simulink model "microgrid_WithBESS"  (R2023a)
settings: Solver=ode23t  StartTime=0.0  StopTime=86000  RelTol=1e-3
PreLoadFcn:
  | addpath('Resources')
InitFcn:
  | initialConditions();
values from neighbouring files (symbols this model uses):
  battEnergy = 3.6e6*BattCap    (= 2059200000)    [initialConditions.m]
  optTime = timeOptimize*60    (= 300)    [initialConditions.m]
libraries: simulink x8, spsThreePhaseDynamicLoadLib x3, spsPower3phPhasorLib x3, spsThreePhaseVIMeasurementLib x3, spsThreePhaseBreakerLib x3, spsThreePhaseSourceLib x2, spsThreePhasePISectionLineLib x1, spsThreePhaseSeriesRLCLoadLib x1, powerlib_meascontrol x1, powerlib x1, spsFrequencyPhasorLib x1, spsSequenceAnalyzerPhasorLib x1
settings Model: Creator=jlesage  LastModifiedBy=KeronDenny
settings SolverCC: AlgebraicLoopSolver=TrustRegion
settings DataIOCC: ReturnWorkspaceOutputs=off
settings DebuggingCC: PregeneratedLibrarySubsystemCodeDiagnostic=none  ArithmeticOperatorsInVariantConditions=warning
settings ModelReferenceCC: EnableRefExpFcnMdlSchedulingChecks=on
settings SFSimCC: SimUseLocalCustomCode=off  CustomCodeUndefinedFunction=UseInterfaceOnly
settings RTWCC: RTWUseLocalCustomCode=off

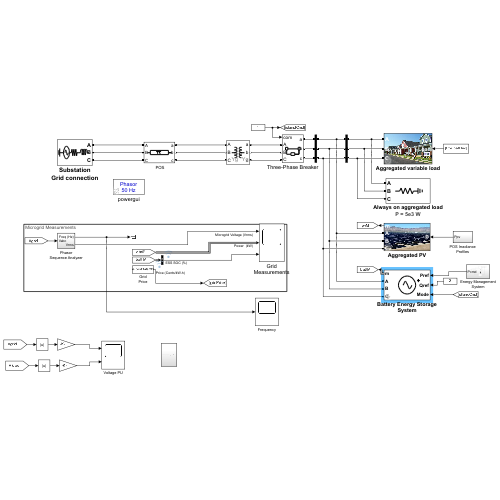
[thumbnail: Simulink's stored preview of the top-level diagram]
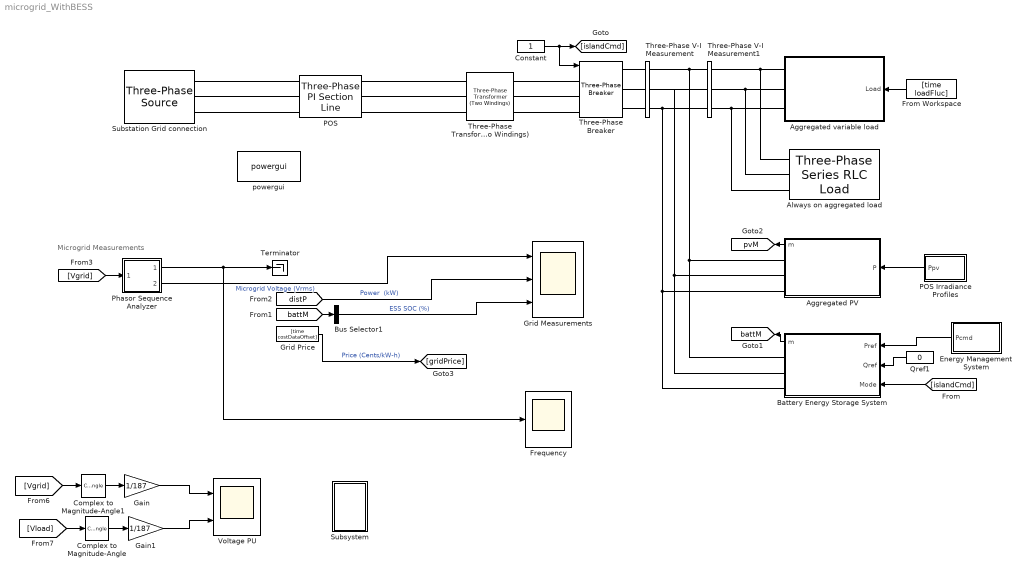
== system microgrid_WithBESS ==
  note: Microgrid Measurements
  " POS " : spsThreePhasePISectionLineLib/Three-Phase PI Section Line  LConnTagsString=a|b|c  RConnTagsString=A|B|C  Length=1.18  Frequency=50  Resistances=[60.9 0.001]  Inductances="[3.52e-2  3.483e-3]"  Capacitances="[ 11.09729e-09   4.8118e-09]"
  Aggregated PV : Subsystem  mask(Grid-Connected PV Array (PQ Model)){Vn=230, Fn=50, P0=400e3}
      mask prompts: Vn "Nominal L-L Voltage [Vrms]"; Fn "Nominal Frequency [Hz]"; P0 "Initial Power [W]"
      mask help:
      | This block models a grid-connected solar array using the Three-Phase Dynamic Load block. This is a system-level model that does not contain any power electronics, but is useful for load flow, phasor, and hybrid phasor-EMT simulations. The input to this block is the power output of the grid connected PV array, not irradiance.
      |
      | For more detailed PV models, consider the PV Array block in the Renewables library. Consider using this PQ Model to perform load flow studies and switch to a more detailed model when full EMT studies are required.
      |
      | Note: The array power must be specified for use for Load Flow analysis.
      mask init:
      | % P0 = Irr0*TotalArea*Efficiency/100;
      | P0 = -P0;
      mask Display:
      | image(imread('PV_Farm.jpg'))
      | color('white')
      | port_label('input',1,'P')
      | port_label('output',1,'m')
      | port_label('Rconn',1,'A')
      | port_label('Rconn',2,'B')
      | port_label('Rconn',3,'C')
  Aggregated variable load : Subsystem  mask(Variable Load (PQ Model)){Vn=230, Fn=50, PF=1, Load0=10e3}
      mask prompts: Vn "Nominal L-L Voltage [Vrms]"; Fn "Nominal Frequency [Hz]"; PF "Power Factor [0 to 1]"; Load0 "Initial Load [W]"
      mask help:
      | The Variable Load block is a lumped approximation for a distribution feeder. For non-unity power factor loads, the input (active power) is scaled accordingly to generate a desired load.
      |
      | Note: The initial input load must be specified for use for Load Flow analysis.
      mask init:
      | P0 = Load0;
      | Q0 = Load0*sqrt(1/PF^2-1);
      mask Display:
      | image(imread('Residential.jpg'))
      | color('white')
      | port_label('input',1,'Load')
      | port_label('Rconn',1,'A')
      | port_label('Rconn',2,'B')
      | port_label('Rconn',3,'C')
  Always on aggregated load : spsThreePhaseSeriesRLCLoadLib/Three-Phase Series RLC Load  LConnTagsString=A|B|C  Configuration=Y (grounded)  NominalVoltage=230  Vabc=[1e3 1e3 1e3]  Vabcp=[1e3 1e3 1e3]  NominalFrequency=50  UnbalancedPower=off  ActivePower=5e3  InductivePower=0  CapacitivePower=0  Pabc=[10e3 9e3 11e3]  QLabc=[100 90 110]  QCabc=[100 90 110]  Pabcp=[10e3 9e3 11e3]  QLabcp=[100 90 110]  QCabcp=[100 90 110]  Measurements=None  LoadType=constant Z
      settings: AttributesFormatString=P = %<ActivePower> W
  Battery Energy Storage System : Subsystem  mask(Grid-connected Energy Storage (PQ Model)){SimMode=Phasor, Vn=230, Fn=50, PnomkW=143, kWh_Rated=572, Efficiency=96, LimitVec=[79 21], RechargeSOC=12, Precharge=100, autoRecharge=on, Initial_kWh_pc=21, PQvec=[400e3 0]}
      mask prompts: SimMode "Simulation Mode"; Vn "Nominal L-L Voltage [Vrms]"; Fn "Nominal Frequency [Hz]"; PnomkW "Rated Power [kW]"; kWh_Rated "Rated Capacity [kWh]"; Efficiency "Overall System Efficiency [%]"; LimitVec "Upper/Lower Charge Limits [%]"; RechargeSOC "SOC to Recharge [%]"; Precharge "Recharge Rate [% of Rated Power]"; autoRecharge "Enable Auto-Recharge"; Initial_kWh_pc "Initial State-of-Charge [0-100%]"; PQvec "Initial Active/Reactive Cmds"
      mask help:
      | The energy storage block models a generic grid-connected energy storage system (ESS), most commonly a battery system. This is a system-level model that does not contain any power electronics, but is useful for load flow, phasor, and hybrid phasor-EMT simulations. The inputs to this block are the commanded active and reactive power of the ESS. The ESS is assumed to have four quadrent operation. The Mode Input dictates what high-level operation the ESS has: current control (Mode = 1) or voltage control (Mode = 0). Current control is ideal for a grid connected system where you need to specify P,Q commands. Voltage control is necessary if the ESS will be the only system supporting the microgrid in islanded mode.
      |
      | For more detailed ESS models, consider the battery block in the Drives library. Consider using this PQ Model to perform load flow studies and switch to a more detailed model when full EMT studies or more advanced controls are required.
      |
      | Note: The initial active/reactive power commands must be specified for use for Load Flow analysis.
      mask init:
      | % Calculate Initial Conditions
      | Pnom = PnomkW*1e3;
      | P0 = -PQvec(1);  Q0 = -PQvec(2);
      | if abs(P0) > Pnom
      |     P0 = sign(P0)*Pnom;
      | end
      | 
      | % Calculate Q0 given Reactive Power Capability Curve
      | Qlim = sqrt(Pnom^2 - P0^2);
      | if Qlim > abs(Q0)
      |     Q0 = sign(Q0)*Qlim;
      | end
      | 
      | UpChrgLim = LimitVec(1);
      | LowChrgLim = LimitVec(2);
      | if Initial_kWh_pc > UpChrgLim && P0 < 0
      |     P0 = 0; Q0 = 0;
      | elseif Initial_kWh_pc < LowChrgLim && P0 > 0
      |     P0 = 0; Q0 = 0;
      | end
      | 
      | simulationStatus =  get_param(bdroot,'SimulationStatus');
      | 
      | % The active variant can only be modified at edit-time or very early during
      | % the simulink compile stage. 
      | if any(strcmp(simulationStatus, {'stopped'}))
      | 
      | blk = [gcb '/Power Measures'];
      | if strcmp(SimMode,'Phasor')
      |     set_param(blk,'OverrideUsingVariant','Phasor');
      | else
      |     set_param(blk,'OverrideUsingVariant','EMT');
      | end
      | 
      | 
      | end
      mask TypeOptions SimMode: Electromagnetic Transient (EMT) | Phasor
      mask DialogControl Container7 Prompt: Grid Connection Properties
      mask DialogControl Container11 Prompt: Charge/Discharge Controls
      mask DialogControl Container12 Prompt: Initial Conditions
      mask Display: plot(-80,-50,80,50,[0,9,18,24,29,30,29,24,18,9,0,-9,-18,-24,-29,-30,-29,-24,-18,-9,0],[30,29,24,18,9,0,-9,-18,-24,-29,-30,-29,-24,-18,-9,0,9,18,24,29,30],[-50],[0],[50],[0],[45 35 40 40 40],[15 15 15 20 10],[1 2 3 4 5 6 7 8 9 10 11 12 13 14 15 16 17 18 19 20 21].*1.5-15,[0,9,18,24,29,30,29,24,18,9,0,-9,-18,-24,-29,-30,-29,-24,-18,-9,0]./2.4)
  Bus Selector1 : BusSelector  OutputSignals=SOC (%)  OutputAsBus=on
  Complex to Magnitude-Angle : ComplexToMagnitudeAngle  Output=Magnitude
  Complex to Magnitude-Angle1 : ComplexToMagnitudeAngle  Output=Magnitude
  Constant : Constant
  Energy Management System : Subsystem
  Frequency : Scope
  From Workspace : FromWorkspace  VariableName=[time loadFluc]
  Gain : Gain  Gain=1/187
  Gain1 : Gain  Gain=1/187
  Grid Measurements : Scope  NumInputPorts=3
  Grid Price : FromWorkspace  VariableName=[time costDataOffset]
  POS Irradiance Profiles : Subsystem
  Phasor Sequence Analyzer : Subsystem
  Qref1 : Constant  Value=0
  Substation Grid connection : spsThreePhaseSourceLib/Three-Phase Source  InternalConnection=Yg  VoltagePhases=off  Voltage=(11000)*1  PhaseAngle=0.071468  Voltage_phases=[25e3 25e3 25e3]/sqrt(3)  PhaseAngles_phases=[0 -120 +120]  Frequency=50  NonIdealSource=on  SpecifyImpedance=on  Resistance=0.8929  Inductance=16.58e-3  ShortCircuitLevel=200e3  BaseVoltage=230  XRratio=0.07  BusType=swing  Pref=10e3  Qref=0  Prefabc=[10e3, 10e3, 10e3]  Qrefabc=[0, 0, 0]  Qmin=-inf  Qmax=inf
  Subsystem : Subsystem
  Terminator : Terminator
  Three-Phase Transformer (Two Windings) : spsThreePhaseTransformerTwoWindingsLib/Three-Phase Transformer (Two Windings)  Winding1Connection=Yg  Winding2Connection=Yg  CoreType=Three single-phase transformers  SetSaturation=off  Hysteresis=off  DataFile='hysteresis'  SetInitialFlux=off  Measurements=None  UNITS=pu  NominalPower=[200e3, 50 ]  Winding1=[ 11e3 , 0.002 , 0.08 ]  Winding2=[ 230 , 0.002 , 0.08 ]  Rm=500  Lm=500  L0=0.5  Saturation=[ 0,0 ; 0.0024,1.2 ; 1.0,1.52 ]  InitialFluxes=[ 0.8 , -0.8 , 0.7 ]  BreakLoop=off  DiscreteSolver=Trapezoidal iterative  DataType=off  TransfoNumber=1
  Three-Phase V-I Measurement : spsThreePhaseVIMeasurementLib/Three-Phase V-I Measurement  VoltageMeasurement=phase-to-ground  SetLabelV=on  LabelV=Vgrid  Vpu=off  VpuLL=off  CurrentMeasurement=yes  SetLabelI=on  LabelI=Igrid  Ipu=off  Pbase=100e6  Vbase=500e3  OutputType=Complex  PhasorSimulation=on  PSBequivalent=0
  Three-Phase V-I Measurement1 : spsThreePhaseVIMeasurementLib/Three-Phase V-I Measurement  VoltageMeasurement=phase-to-ground  SetLabelV=on  LabelV=Vload  Vpu=off  VpuLL=off  CurrentMeasurement=yes  SetLabelI=on  LabelI=Iload  Ipu=off  Pbase=100e6  Vbase=500e3  OutputType=Complex  PhasorSimulation=on  PSBequivalent=0
  Three-Phase Breaker : spsThreePhaseBreakerLib/Three-Phase Breaker  InitialState=closed  SwitchA=on  SwitchB=on  SwitchC=on  SwitchTimes="[1/60  5/60]"  External=on  BreakerResistance=0.01  SnubberResistance=1e6  SnubberCapacitance=inf  Measurements=None
  Voltage PU : Scope  NumInputPorts=2
  powergui : sps_lib/powergui  Priority=1  SimulationMode=Phasor  SampleTime=1e-4  frequency=50  Iterations=50  frequencyindice=50  Pbase=100e6  ErrMax=0.0001  UnitsV=kV  UnitsW=MW  buscounter=3  FunctionMessages=off  echomessages=off  EnableUseOfTLC=off  CurrentSourceSwitches=off  DisableSnubberDevices=off  DisableRonSwitches=off  DisableVfSwitches=off  DisplayEquations=off  AutomaticDiscreteSolvers=off  SolverType=Tustin/Backward Euler (TBE)  Interpol=off  ExternalGateDelay=off  methode=off  Ts=100  x0status=blocks  SPID=on  SwTol=0  HookPort=off  NonlinearTolerance=0  nMaxIteration=15  ContinueOnMaxIteration=off  RestoreLinks=warning  ResistiveCurrentMeasurement=off  Frange=[0:2:500]  Ylog=off  Xlog=on  ShowGrid=off  save=off  variable=ZData  structure=0  ZoomFFT=off  StartTime=0.0  cycles=1  DisplayStyle=1  fundamental=60  FreqAxis=off  MaxFrequency=1000  frequencyindicesteady=1  RmsSteady=1  display=off
  tag scope: battM=global, pvM=global
  wires:
  Qref1/1 -> Battery Energy Storage System/2(Qref)
  Battery Energy Storage System/1(m) -> [battM]
  Aggregated PV/1(m) -> [pvM]
  [Vgrid] -> Phasor Sequence Analyzer/1(Vabc)
  [islandCmd] -> Battery Energy Storage System/3(Mode)
  Constant/1 -> [islandCmd], Three-Phase Breaker/1
  [distP] -> Grid Measurements/2  "Power  (kW)"
  Phasor Sequence Analyzer/2(Vrms) -> Grid Measurements/1  "Microgrid Voltage (Vrms)"
  [battM] -> Bus Selector1/1
  Phasor Sequence Analyzer/1(Freq (Hz)) -> Terminator/1, Frequency/1
  Grid Price/1 -> [gridPrice]  "Price (Cents/kW-h)"
  [Vload] -> Complex to Magnitude-Angle/1
  [Vgrid] -> Complex to Magnitude-Angle1/1
  Complex to Magnitude-Angle/1 -> Gain1/1
  Complex to Magnitude-Angle1/1 -> Gain/1
  Gain/1 -> Voltage PU/1
  Gain1/1 -> Voltage PU/2
  Bus Selector1/1 -> Grid Measurements/3  "ESS SOC (%)"
  Energy Management System/1(Pcmd) -> Battery Energy Storage System/1(Pref)
  POS Irradiance Profiles/1(Ppv) -> Aggregated PV/1(P)
  From Workspace/1 -> Aggregated variable load/1(Load)
  connections:
  " POS "/RConn1 -- Three-Phase Transformer (Two Windings)/LConn1
  " POS "/RConn2 -- Three-Phase Transformer (Two Windings)/LConn2
  " POS "/RConn3 -- Three-Phase Transformer (Two Windings)/LConn3
  Three-Phase Transformer (Two Windings)/RConn1 -- Three-Phase Breaker/LConn1
  Three-Phase Transformer (Two Windings)/RConn2 -- Three-Phase Breaker/LConn2
  Three-Phase Transformer (Two Windings)/RConn3 -- Three-Phase Breaker/LConn3
  Always on aggregated load/LConn2 -- Aggregated variable load/RConn2 -- Three-Phase V-I Measurement1/RConn2
  Three-Phase V-I Measurement/RConn3 -- Three-Phase V-I Measurement1/LConn3 -- Battery Energy Storage System/RConn3 -- Aggregated PV/RConn3
  Three-Phase Breaker/RConn1 -- Three-Phase V-I Measurement/LConn1
  Three-Phase Breaker/RConn2 -- Three-Phase V-I Measurement/LConn2
  Three-Phase Breaker/RConn3 -- Three-Phase V-I Measurement/LConn3
  Always on aggregated load/LConn1 -- Aggregated variable load/RConn1 -- Three-Phase V-I Measurement1/RConn1
  Three-Phase V-I Measurement/RConn1 -- Three-Phase V-I Measurement1/LConn1 -- Battery Energy Storage System/RConn1 -- Aggregated PV/RConn1
  Battery Energy Storage System/RConn2 -- Three-Phase V-I Measurement/RConn2 -- Three-Phase V-I Measurement1/LConn2 -- Aggregated PV/RConn2
  Always on aggregated load/LConn3 -- Aggregated variable load/RConn3 -- Three-Phase V-I Measurement1/RConn3
  Substation Grid connection/RConn1 -- " POS "/LConn1
  Substation Grid connection/RConn2 -- " POS "/LConn2
  Substation Grid connection/RConn3 -- " POS "/LConn3

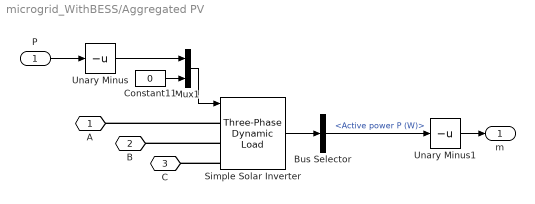
== system microgrid_WithBESS/Aggregated PV ==
  P : Inport
  Bus Selector : BusSelector  OutputSignals=Active power P (W)
  Constant11 : Constant  Value=0
  Mux1 : Mux  Inputs=2
  Simple Solar Inverter : spsThreePhaseDynamicLoadLib/Three-Phase Dynamic Load  NominalVoltage=[Vn Fn]  ActiveReactivePowers=[-250000 -3.38813e-13]  PositiveSequence=[0.999844 -0.0038635]  ExternalControl=on  NpNq=[1.3 2]  TimeConstants="[0  0  0  0]"  MinimumVoltage=0.7  Tfilter=1e-2  LoadFlowParameters=[4,0,0,0,0]
      settings: LibrarySourceBlock=|
      | sps_lib/Passives/Three-Phase
      | Dynamic Load
  Unary Minus : UnaryMinus
  Unary Minus1 : UnaryMinus
  A : PMIOPort  Side=Right
  B : PMIOPort  Port=2  Side=Right
  C : PMIOPort  Port=3  Side=Right
  m : Outport  VectorParamsAs1DForOutWhenUnconnected=off
  wires:
  P/1 -> Unary Minus/1
  Unary Minus/1 -> Mux1/1
  Mux1/1 -> Simple Solar Inverter/1
  Constant11/1 -> Mux1/2
  Simple Solar Inverter/1 -> Bus Selector/1
  Bus Selector/1 -> Unary Minus1/1  "<Active power P (W)>"
  Unary Minus1/1 -> m/1
  connections:
  Simple Solar Inverter/LConn2 -- B/RConn1
  Simple Solar Inverter/LConn3 -- C/RConn1
  Simple Solar Inverter/LConn1 -- A/RConn1

== system microgrid_WithBESS/Aggregated variable load ==
  Load : Inport
  Dynamic Load Control : Subsystem
  Simple Three-Phase Load : spsThreePhaseDynamicLoadLib/Three-Phase Dynamic Load  NominalVoltage=[Vn Fn]  ActiveReactivePowers=[200000 45883.1]  PositiveSequence=[0.999844 -0.0038635]  ExternalControl=on  NpNq=[1.3 2]  TimeConstants="[0  0  0  0]"  MinimumVoltage=0.7  Tfilter=1e-2  LoadFlowParameters=[4,0,0,0,0]
      settings: LibrarySourceBlock=|
      | sps_lib/Passives/Three-Phase
      | Dynamic Load
  Terminator : Terminator
  A : PMIOPort  Side=Right
  B : PMIOPort  Port=2  Side=Right
  C : PMIOPort  Port=3  Side=Right
  wires:
  Simple Three-Phase Load/1 -> Terminator/1
  Load/1 -> Dynamic Load Control/1(P0)
  Dynamic Load Control/1(PQ) -> Simple Three-Phase Load/1
  connections:
  Simple Three-Phase Load/LConn1 -- A/RConn1
  Simple Three-Phase Load/LConn3 -- C/RConn1
  Simple Three-Phase Load/LConn2 -- B/RConn1

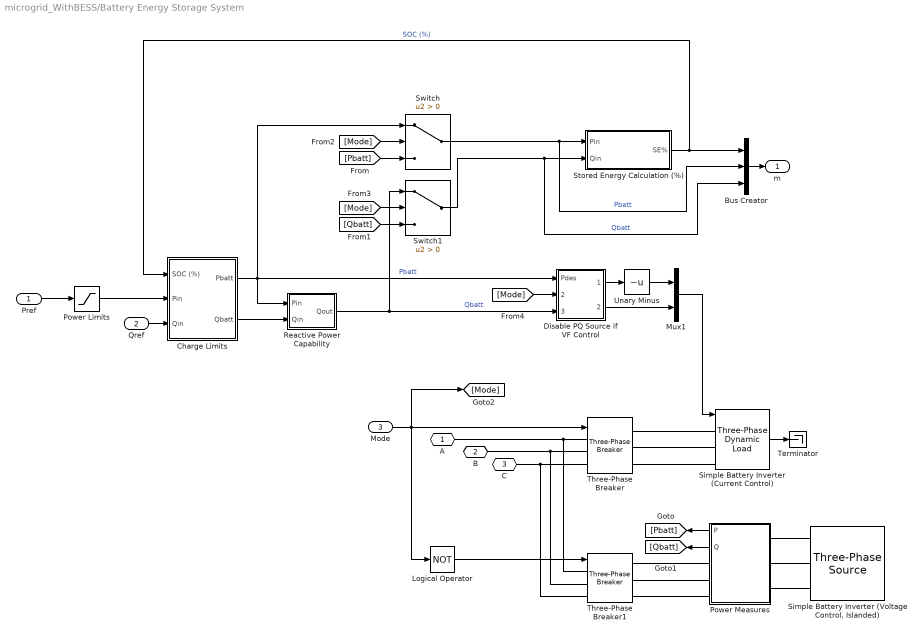
== system microgrid_WithBESS/Battery Energy Storage System ==
  Pref : Inport
  Qref : Inport  Port=2
  Mode : Inport  Port=3
  Bus Creator : BusCreator  Inputs=3
  Charge Limits : Subsystem
  Disable PQ Source if VF Control : Subsystem
  Logical Operator : Logic  Operator=NOT  AllPortsSameDT=off  OutDataTypeStr=boolean
  Mux1 : Mux  Inputs=2
  Power Limits : Saturate  UpperLimit=Pnom  LowerLimit=-Pnom
  Power Measures : Subsystem  Variant=on  VariantControlMode=label  LabelModeActiveChoice=Phasor
  Reactive Power Capability : Subsystem
  Simple Battery Inverter (Current Control) : spsThreePhaseDynamicLoadLib/Three-Phase Dynamic Load  NominalVoltage=[Vn Fn]  ActiveReactivePowers=[-100e3 -3.38813e-13]  PositiveSequence=[0.999844 -0.0038635]  ExternalControl=on  NpNq=[1.3 2]  TimeConstants="[0  0  0  0]"  MinimumVoltage=0.7  Tfilter=1e-2  LoadFlowParameters=[4,0,0,0,0]
      settings: LibrarySourceBlock=|
      | sps_lib/Passives/Three-Phase
      | Dynamic Load
  "Simple Battery Inverter (Voltage Control, Islanded)" : spsThreePhaseSourceLib/Three-Phase Source  InternalConnection=Yg  VoltagePhases=off  Voltage=Vn  PhaseAngle=0  Voltage_phases=[25e3 25e3 25e3]/sqrt(3)  PhaseAngles_phases=[0 -120 +120]  Frequency=Fn  NonIdealSource=off  SpecifyImpedance=off  Resistance=0.8929  Inductance=16.58e-3  ShortCircuitLevel=100e6  BaseVoltage=25e3  XRratio=7  BusType=swing  Pref=10e3  Qref=0  Prefabc=[10e3, 10e3, 10e3]  Qrefabc=[0, 0, 0]  Qmin=-inf  Qmax=inf
  Stored Energy Calculation (%) : Subsystem
  Switch : Switch  Criteria=u2 > Threshold  SaturateOnIntegerOverflow=off  InputSameDT=off
  Switch1 : Switch  Criteria=u2 > Threshold  SaturateOnIntegerOverflow=off  InputSameDT=off
  Terminator : Terminator
  Three-Phase Breaker : spsThreePhaseBreakerLib/Three-Phase Breaker  InitialState=closed  SwitchA=on  SwitchB=on  SwitchC=on  SwitchTimes="[1/60  5/60]"  External=on  BreakerResistance=0.01  SnubberResistance=1e6  SnubberCapacitance=inf  Measurements=None
  Three-Phase Breaker1 : spsThreePhaseBreakerLib/Three-Phase Breaker  InitialState=open  SwitchA=on  SwitchB=on  SwitchC=on  SwitchTimes="[1/60  5/60]"  External=on  BreakerResistance=0.01  SnubberResistance=1e6  SnubberCapacitance=inf  Measurements=None
  Unary Minus : UnaryMinus
  A : PMIOPort  Side=Right
  B : PMIOPort  Port=2  Side=Right
  C : PMIOPort  Port=3  Side=Right
  m : Outport  VectorParamsAs1DForOutWhenUnconnected=off
  wires:
  Charge Limits/2(Qbatt) -> Reactive Power Capability/2(Qin)
  Qref/1 -> Charge Limits/3(Qin)
  Power Limits/1 -> Charge Limits/2(Pin)
  Stored Energy Calculation (%)/1(SE%) -> Bus Creator/1, Charge Limits/1(SOC (%))  "SOC (%)"
  Bus Creator/1 -> m/1
  Pref/1 -> Power Limits/1
  Simple Battery Inverter (Current Control)/1 -> Terminator/1
  Mux1/1 -> Simple Battery Inverter (Current Control)/1
  Unary Minus/1 -> Mux1/1
  Logical Operator/1 -> Three-Phase Breaker1/1
  Mode/1 -> [Mode], Logical Operator/1, Three-Phase Breaker/1
  Power Measures/1(P) -> [Pbatt]
  Power Measures/2(Q) -> [Qbatt]
  Switch/1 -> Bus Creator/2, Stored Energy Calculation (%)/1(Pin)  "Pbatt"
  Switch1/1 -> Bus Creator/3, Stored Energy Calculation (%)/2(Qin)  "Qbatt"
  [Mode] -> Switch/2
  [Mode] -> Switch1/2
  [Qbatt] -> Switch1/3
  [Pbatt] -> Switch/3
  Charge Limits/1(Pbatt) -> Switch/1, Reactive Power Capability/1(Pin), Disable PQ Source if VF Control/1(Pdes)  "Pbatt"
  [Mode] -> Disable PQ Source if VF Control/2(Mode)
  Reactive Power Capability/1(Qout) -> Disable PQ Source if VF Control/3(Qdes), Switch1/1  "Qbatt"
  Disable PQ Source if VF Control/1(Pbatt) -> Unary Minus/1
  Disable PQ Source if VF Control/2(Qbatt) -> Mux1/2
  connections:
  Three-Phase Breaker/RConn1 -- Simple Battery Inverter (Current Control)/LConn1
  Three-Phase Breaker/RConn2 -- Simple Battery Inverter (Current Control)/LConn2
  Three-Phase Breaker/RConn3 -- Simple Battery Inverter (Current Control)/LConn3
  Three-Phase Breaker/LConn3 -- Three-Phase Breaker1/LConn3 -- C/RConn1
  Three-Phase Breaker/LConn2 -- B/RConn1 -- Three-Phase Breaker1/LConn2
  Three-Phase Breaker/LConn1 -- A/RConn1 -- Three-Phase Breaker1/LConn1
  Power Measures/LConn1 -- "Simple Battery Inverter (Voltage Control, Islanded)"/RConn1
  Power Measures/RConn1 -- Three-Phase Breaker1/RConn1
  Power Measures/LConn2 -- "Simple Battery Inverter (Voltage Control, Islanded)"/RConn2
  Power Measures/RConn2 -- Three-Phase Breaker1/RConn2
  Power Measures/LConn3 -- "Simple Battery Inverter (Voltage Control, Islanded)"/RConn3
  Power Measures/RConn3 -- Three-Phase Breaker1/RConn3

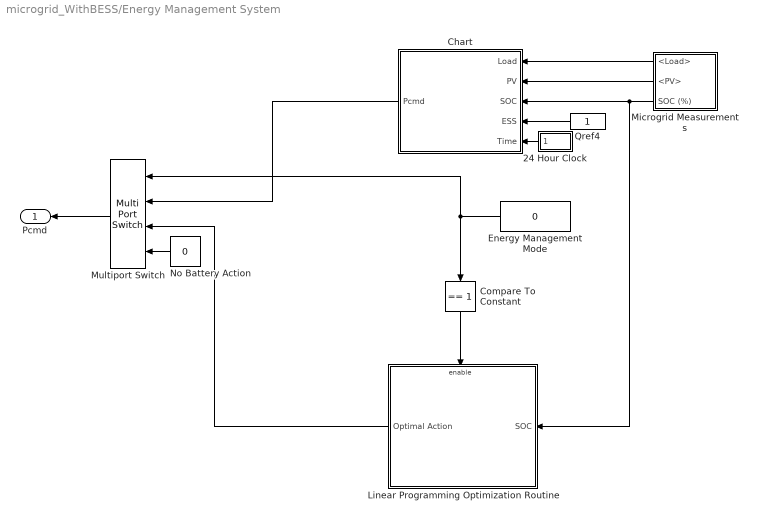
== system microgrid_WithBESS/Energy Management System ==
  24 Hour Clock : Subsystem
  Chart : Stateflow chart  TreatAsAtomicUnit=on  SystemSampleTime=360
  Compare To Constant : simulink/Logic and Bit Operations/Compare To Constant  relop===  const=1  OutDataTypeStr=boolean
  Energy Management Mode : Constant  Value=0
  Linear Programming Optimization Routine : Subsystem  TreatAsAtomicUnit=on
  Microgrid Measurements : Subsystem
  Multiport Switch : MultiPortSwitch  DataPortOrder=Zero-based contiguous  zeroidx=on  SaturateOnIntegerOverflow=off  InputSameDT=off
  No Battery Action : Constant  Value=0
  Qref4 : Constant
  Pcmd : Outport  VectorParamsAs1DForOutWhenUnconnected=off
  wires:
  Microgrid Measurements/1(<Load>) -> Chart/1(Load)
  24 Hour Clock/1(Time) -> Chart/5(Time)
  Microgrid Measurements/2(<PV>) -> Chart/2(PV)
  Microgrid Measurements/3(SOC (%)) -> Chart/3(SOC), Linear Programming Optimization Routine/1(SOC)
  Qref4/1 -> Chart/4(ESS)
  Multiport Switch/1 -> Pcmd/1
  Chart/1(Pcmd) -> Multiport Switch/2
  Energy Management Mode/1 -> Multiport Switch/1, Compare To Constant/1
  Linear Programming Optimization Routine/1(Optimal Action) -> Multiport Switch/3
  Compare To Constant/1 -> Linear Programming Optimization Routine/Enable
  No Battery Action/1 -> Multiport Switch/4

== system microgrid_WithBESS/POS Irradiance Profiles ==
  From Workspace1 : FromWorkspace  VariableName=[time cloudyPpv]
  From Workspace2 : FromWorkspace  VariableName=[time clearPpv]
  Profile Select : Constant  Value=0
  Switch : Switch  Criteria=u2 > Threshold  SaturateOnIntegerOverflow=off  InputSameDT=off
  Ppv : Outport  VectorParamsAs1DForOutWhenUnconnected=off
  wires:
  From Workspace2/1 -> Switch/1
  Profile Select/1 -> Switch/2, [PVDay]
  From Workspace1/1 -> Switch/3
  Switch/1 -> Ppv/1

== system microgrid_WithBESS/Phasor Sequence Analyzer ==
  Vabc : Inport
  Frequency (Phasor) : spsFrequencyPhasorLib/Frequency (Phasor)  Fn=50  T=0.1
      settings: LibrarySourceBlock=|
      | sps_lib/Sensors and Measurements/Frequency
      | (Phasor)
  LG to LL : Gain  Gain=sqrt(3)/sqrt(2)
  Sequence Analyzer (Phasor) : spsSequenceAnalyzerPhasorLib/Sequence Analyzer (Phasor)  seq=Positive
      settings: LibrarySourceBlock=|
      | sps_lib/Sensors and Measurements/Sequence Analyzer
      | (Phasor)
  Terminator : Terminator
  deg-to-rad : Gain  Gain=pi/180
  Freq (Hz) : Outport  VectorParamsAs1DForOutWhenUnconnected=off
  Vrms : Outport  Port=2  VectorParamsAs1DForOutWhenUnconnected=off
  wires:
  Sequence Analyzer (Phasor)/1 -> LG to LL/1
  Vabc/1 -> Sequence Analyzer (Phasor)/1
  Sequence Analyzer (Phasor)/2 -> deg-to-rad/1
  deg-to-rad/1 -> Frequency (Phasor)/1
  Frequency (Phasor)/1 -> Freq (Hz)/1
  Frequency (Phasor)/2 -> Terminator/1
  LG to LL/1 -> Vrms/1

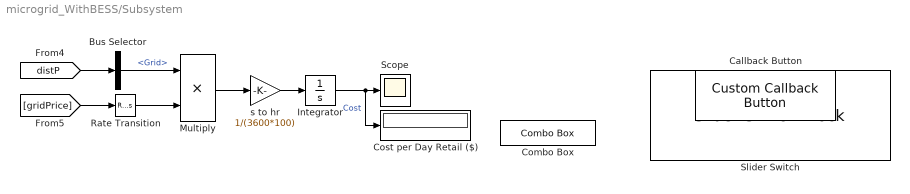
== system microgrid_WithBESS/Subsystem ==
  Bus Selector : BusSelector  OutputSignals=Grid
  Callback Button : CustomCallbackButton  Configuration="{\"components\":[{\"name\":\"BackgroundImageComponent\",\"settings\":{\"image\":{\"size\":[0,0],\"src\":\"default\",\"srcOrientation\":\"Right\"},\"position\":[0,0,1,1]}},{\"name\":\"ButtonStateComponent\",\"settings\":{\"buttonType\":\"momentary\",\"clickFcn\":\"compareCosts();\",\"onValue\":1,\"position\":[0,0,1,1],\"pressDelay\":\"500\",\"pressFcn\":\"\",\"repeatInterval\":\"0\",\"states\":[{\"horizontalAlignment\":\"center\",\"image\":{\"position\":[0,0,1,1],\"src\":\"default\",\"srcOrientation\":\"Right\"},\"label\":{\"color\":[0.01176470588,0.01176470588,0.01176470588,1],\"icon\":{\"size\":[0,0],\"src\":\"default\",\"srcOrientation\":\"Right\"},\"iconPlacement\":\"left\",\"text\":{\"content\":\"Compare Methods\"}},\"labelOffset\":[0,0],\"verticalAlignment\":\"middle\"},{\"horizontalAlignment\":\"center\",\"image\":{\"position\":[0,0,1,1],\"src\":\"default\",\"srcOrientation\":\"Right\"},\"label\":{\"color\":[0.01176470588,0.01176470588,0.01176470588,1],\"icon\":{\"size\":[0,0],\"src\":\"default\",\"srcOrientation\":\"Right\"},\"iconPlacement\":\"left\",\"text\":{\"content\":\"Compare Methods\"}},\"labelOffset\":[0,0],\"verticalAlignment\":\"middle\"},{\"horizontalAlignment\":\"center\",\"image\":{\"position\":[0,0,1,1],\"src\":\"default\",\"srcOrientation\":\"Right\"},\"label\":{\"color\":[0.01176470588,0.01176470588,0.01176470588,1],\"icon\":{\"size\":[0,0],\"src\":\"default\",\"srcOrientation\":\"Right\"},\"iconPlacement\":\"left\",\"text\":{\"content\":\"Compare Methods\"}},\"labelOffset\":[0,0],\"verticalAlignment\":\"middle\"},{\"horizontalAlignment\":\"center\",\"image\":{\"position\":[0,0,1,1],\"src\":\"default\",\"srcOrientation\":\"Right\"},\"label\":{\"color\":[0.01176470588,0.01176470588,0.01176470588,1],\"icon\":{\"size\":[0,0],\"src\":\"default\",\"srcOrientation\":\"Right\"},\"iconPlacement\":\"left\",\"text\":{\"content\":\"Compare Methods\"}},\"labelOffset\":[0,0],\"verticalAlignment\":\"middle\"}]}},{\"name\":\"ForegroundImageComponent\",\"settings\":{\"image\":{\"size\":[0,0],\"src\":\"default\",\"srcOrientation\":\"Right\"},\"isForeground\":1,\"position\":[0,0,1,1]}}],\"settings\":{\"BindingType\":\"standalone\",\"backgroundColor\":[244,244,244,1],\"backgroundOffset\":0.2,\"backgroundOpacity\":1,\"fixedAspectRatio\":\"off\",\"foregroundColor\":[0.01176470588,0.01176470588,0.01176470588,1],\"migratedFromLegacy\":true,\"useBackgroundColor\":true,\"variant\":\"callback\",\"version\":\"R2023a\"},\"type\":\"Button\"}"  CustomBackgroundColor="{\"color\":[0.9568627451,0.9568627451,0.9568627451],\"show\":true}"
  Combo Box : ComboBox  LabelPosition=Hide  SelectedLabel=Cloudy Day
      settings: Values={{'Clear Day', 'Cloudy Day'}, [1 0]}
  Cost per Day Retail ($) : Display
  Integrator : Integrator
  Multiply : Product
  Rate Transition : RateTransition  OutPortSampleTime=optTime
  Scope : Scope
  Slider Switch : SliderSwitchBlock
      settings: Values={{'Chart', 'Optimization'}, [0 1]}
  s to hr : Gain  Gain=1/(3600*100)
  wires:
  Integrator/1 -> Cost per Day Retail ($)/1, Scope/1  "Cost"
  [gridPrice] -> Rate Transition/1
  Bus Selector/1 -> Multiply/1  "<Grid>"
  Multiply/1 -> s to hr/1
  [distP] -> Bus Selector/1
  Rate Transition/1 -> Multiply/2
  s to hr/1 -> Integrator/1

== system microgrid_WithBESS/Aggregated variable load/Dynamic Load Control ==
  P0 : Inport
  Fcn : Fcn  Expr=sqrt(1/u(1)^2-1)
  Mux : Mux  Inputs=2
  Product : Product
  Summer1 : Constant  Value=PF
  PQ : Outport  VectorParamsAs1DForOutWhenUnconnected=off
  wires:
  Summer1/1 -> Fcn/1
  Fcn/1 -> Product/2
  P0/1 -> Product/1, Mux/1
  Mux/1 -> PQ/1
  Product/1 -> Mux/2  "Qo"

== system microgrid_WithBESS/Battery Energy Storage System/Charge Limits ==
  SOC (%) : Inport
  Pin : Inport  Port=2
  Qin : Inport  Port=3
  Overcharge Check : Subsystem
  Undercharge Check : Subsystem
  Pbatt : Outport  VectorParamsAs1DForOutWhenUnconnected=off
  Qbatt : Outport  Port=2  VectorParamsAs1DForOutWhenUnconnected=off
  wires:
  SOC (%)/1 -> Overcharge Check/1(SOC (%)), Undercharge Check/1(SOC (%))
  Undercharge Check/2(Qout) -> Qbatt/1
  Pin/1 -> Overcharge Check/2(Pin)
  Overcharge Check/1(Pout) -> Undercharge Check/2(Pin)
  Qin/1 -> Overcharge Check/3(Qin)
  Undercharge Check/1(Pout) -> Pbatt/1  "Pbatt"
  Overcharge Check/2(Qout) -> Undercharge Check/3(Qin)

== system microgrid_WithBESS/Battery Energy Storage System/Disable PQ Source if VF Control ==
  Pdes : Inport
  Mode : Inport  Port=2
  Qdes : Inport  Port=3
  Constant : Constant  Value=0
  Constant1 : Constant  Value=0
  Switch2 : Switch  Criteria=u2 > Threshold  SaturateOnIntegerOverflow=off  InputSameDT=off
  Switch3 : Switch  Criteria=u2 > Threshold  SaturateOnIntegerOverflow=off  InputSameDT=off
  Pbatt : Outport  VectorParamsAs1DForOutWhenUnconnected=off
  Qbatt : Outport  Port=2  VectorParamsAs1DForOutWhenUnconnected=off
  wires:
  Mode/1 -> Switch3/2, Switch2/2
  Pdes/1 -> Switch2/1
  Switch2/1 -> Pbatt/1
  Constant1/1 -> Switch3/3
  Switch3/1 -> Qbatt/1
  Constant/1 -> Switch2/3
  Qdes/1 -> Switch3/1

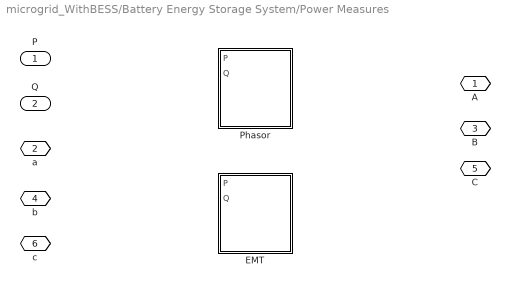
== system microgrid_WithBESS/Battery Energy Storage System/Power Measures ==
  EMT : Subsystem  VariantControl=EMT
  Phasor : Subsystem  VariantControl=Phasor
  A : PMIOPort  Side=Left
  a : PMIOPort  Port=2  Side=Right
  B : PMIOPort  Port=3  Side=Left
  b : PMIOPort  Port=4  Side=Right
  C : PMIOPort  Port=5  Side=Left
  c : PMIOPort  Port=6  Side=Right
  P : Outport  VectorParamsAs1DForOutWhenUnconnected=off
  Q : Outport  Port=2  VectorParamsAs1DForOutWhenUnconnected=off

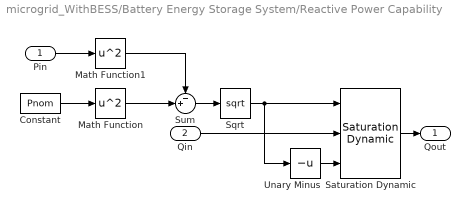
== system microgrid_WithBESS/Battery Energy Storage System/Reactive Power Capability ==
  Pin : Inport
  Qin : Inport  Port=2
  Constant : Constant  Value=Pnom
  Math Function : Math  Operator=square  SignedPower=on
  Math Function1 : Math  Operator=square  SignedPower=on
  Saturation Dynamic : simulink/Discontinuities/Saturation Dynamic  OutMin=[]  OutMax=[]  OutDataTypeStr=Inherit: Same as second input  OutDataType=fixdt(1, 16)  OutScaling=2^-10  DoSatur=off
  Sqrt : Sqrt
  Sum : Sum  Inputs=-+|
  Unary Minus : UnaryMinus
  Qout : Outport  VectorParamsAs1DForOutWhenUnconnected=off
  wires:
  Sqrt/1 -> Saturation Dynamic/1, Unary Minus/1
  Math Function1/1 -> Sum/1
  Math Function/1 -> Sum/2
  Constant/1 -> Math Function/1
  Sum/1 -> Sqrt/1
  Unary Minus/1 -> Saturation Dynamic/3
  Saturation Dynamic/1 -> Qout/1
  Pin/1 -> Math Function1/1
  Qin/1 -> Saturation Dynamic/2

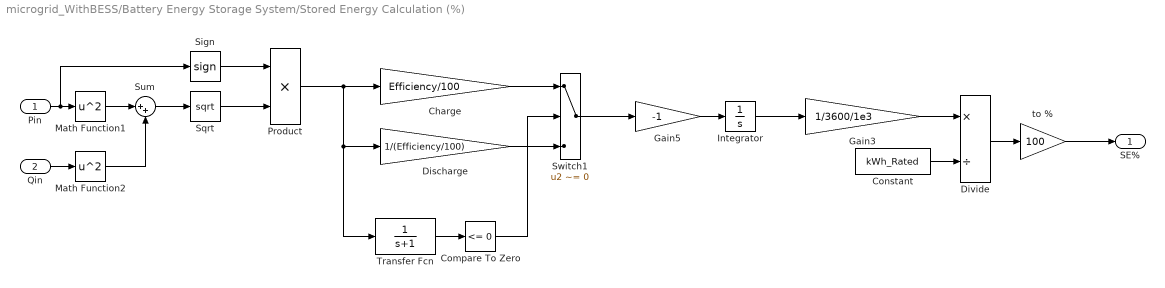
== system microgrid_WithBESS/Battery Energy Storage System/Stored Energy Calculation (%) ==
  Pin : Inport
  Qin : Inport  Port=2
  Charge : Gain  Gain=Efficiency/100
  Compare To Zero : simulink/Logic and Bit Operations/Compare To Zero  relop=<=  OutDataTypeStr=boolean
  Constant : Constant  Value=kWh_Rated
  Discharge : Gain  Gain=1/(Efficiency/100)
  Divide : Product  Inputs=*/
  Gain3 : Gain  Gain=1/3600/1e3
  Gain5 : Gain  Gain=-1
  Integrator : Integrator  InitialCondition=(Initial_kWh_pc/100)*kWh_Rated*3600*1e3
  Math Function1 : Math  Operator=square  SignedPower=on
  Math Function2 : Math  Operator=square  SignedPower=on
  Product : Product
  Sign : Signum
  Sqrt : Sqrt
  Sum : Sum  Inputs=|++
  Switch1 : Switch  Criteria=u2 ~= 0  SaturateOnIntegerOverflow=off  InputSameDT=off
  Transfer Fcn : TransferFcn  Denominator=[1 1]
  to % : Gain  Gain=100
  SE% : Outport  VectorParamsAs1DForOutWhenUnconnected=off
  wires:
  Sign/1 -> Product/1
  Sqrt/1 -> Product/2
  Sum/1 -> Sqrt/1
  Math Function2/1 -> Sum/2
  Math Function1/1 -> Sum/1
  Qin/1 -> Math Function2/1
  Pin/1 -> Math Function1/1, Sign/1
  Product/1 -> Transfer Fcn/1, Discharge/1, Charge/1
  Discharge/1 -> Switch1/3
  Gain5/1 -> Integrator/1
  to %/1 -> SE%/1
  Transfer Fcn/1 -> Compare To Zero/1
  Switch1/1 -> Gain5/1
  Gain3/1 -> Divide/1
  Constant/1 -> Divide/2
  Charge/1 -> Switch1/1
  Divide/1 -> to %/1
  Compare To Zero/1 -> Switch1/2
  Integrator/1 -> Gain3/1

== system microgrid_WithBESS/Energy Management System/24 Hour Clock ==
  Clock : Clock
  Compare To Constant : simulink/Logic and Bit Operations/Compare To Constant  relop=>  const=24*3600  OutDataTypeStr=boolean
  Enabled Subsystem : Subsystem  TreatAsAtomicUnit=on
  Memory : Memory
  Sum : Sum  Inputs=|-+
  to Hours : Gain  Gain=1/3600
  Time : Outport  VectorParamsAs1DForOutWhenUnconnected=off
  wires:
  Sum/1 -> to Hours/1, Memory/1  "Time Elapse"
  Compare To Constant/1 -> Enabled Subsystem/Enable
  Clock/1 -> Enabled Subsystem/1(In1), Sum/2
  Enabled Subsystem/1(Out1) -> Sum/1
  to Hours/1 -> Time/1
  Memory/1 -> Compare To Constant/1

== system microgrid_WithBESS/Energy Management System/Linear Programming Optimization Routine ==
  note: Forecast Algorithms
  SOC : Inport
  Enable : EnablePort
  Nominal Charge : Constant  Value=battEnergy
  Optimization-based Energy Management : MATLAB Function  TreatAsAtomicUnit=on  SystemSampleTime=optTime
  Sliding Cost Values : FromWorkspace  VariableName=CostForecast
  Sliding Load Power : FromWorkspace  VariableName=PloadForecast
  Sliding PV Power : FromWorkspace  VariableName=PpvForecast
  Time between optimizations : Constant  Value=optTime
  Optimal Action : Outport  VectorParamsAs1DForOutWhenUnconnected=off
  wires:
  Optimization-based Energy Management/1(optVec) -> Optimal Action/1
  Time between optimizations/1 -> Optimization-based Energy Management/3(dt)
  Sliding Cost Values/1 -> Optimization-based Energy Management/4(Cost)
  Sliding Load Power/1 -> Optimization-based Energy Management/6(Pload)
  Nominal Charge/1 -> Optimization-based Energy Management/2(Ebatt)
  SOC/1 -> Optimization-based Energy Management/1(SOC)
  Sliding PV Power/1 -> Optimization-based Energy Management/5(Ppv)

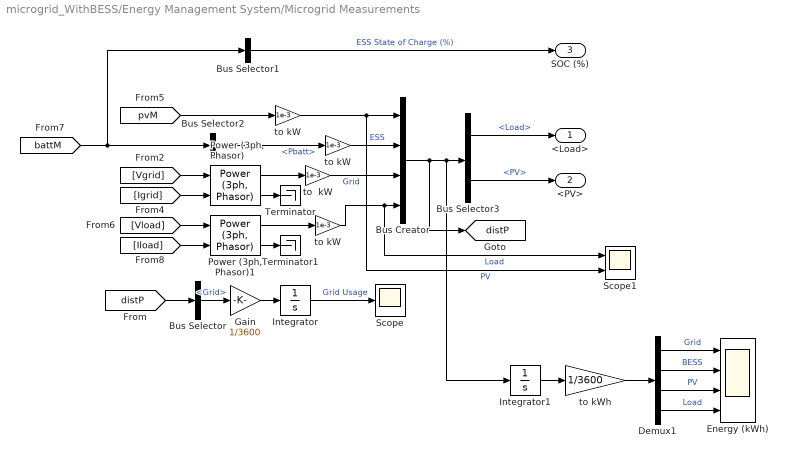
== system microgrid_WithBESS/Energy Management System/Microgrid Measurements ==
  " to kW" : Gain  Gain=1e-3
  Bus Creator : BusCreator  Inputs=4
  Bus Selector : BusSelector  OutputSignals=Grid
  Bus Selector1 : BusSelector  OutputSignals=SOC (%)  OutputAsBus=on
  Bus Selector2 : BusSelector  OutputSignals=Pbatt
  Bus Selector3 : BusSelector  OutputSignals=Load,PV
  Demux1 : Demux
  Energy (kWh) : Scope  NumInputPorts=4
  Gain : Gain  Gain=1/3600
  Integrator : Integrator
  Integrator1 : Integrator
  "Power (3ph, Phasor)" : spsPower3phPhasorLib/Power (3ph, Phasor)
      settings: LibrarySourceBlock=|
      | sps_lib/Sensors and Measurements/Power
      | (3ph, Phasor)
  "Power (3ph, Phasor)1" : spsPower3phPhasorLib/Power (3ph, Phasor)
      settings: LibrarySourceBlock=|
      | sps_lib/Sensors and Measurements/Power
      | (3ph, Phasor)
  Scope : Scope
  Scope1 : Scope  NumInputPorts=2
  Terminator : Terminator
  Terminator1 : Terminator
  to  kW : Gain  Gain=1e-3
  to kW : Gain  Gain=1e-3
  "to kW " : Gain  Gain=1e-3
  to kWh : Gain  Gain=1/3600
  <Load> : Outport  VectorParamsAs1DForOutWhenUnconnected=off
  <PV> : Outport  Port=2  VectorParamsAs1DForOutWhenUnconnected=off
  SOC (%) : Outport  Port=3  VectorParamsAs1DForOutWhenUnconnected=off
  tag scope: distP=global
  wires:
  Bus Creator/1 -> [distP], Integrator1/1, Bus Selector3/1
  "Power (3ph, Phasor)1"/2 -> Terminator1/1
  " to kW"/1 -> Scope1/1, Bus Creator/4  "Load"
  "to kW "/1 -> Bus Creator/2  "ESS"
  [Vload] -> "Power (3ph, Phasor)1"/1
  "Power (3ph, Phasor)"/2 -> Terminator/1
  [pvM] -> to kW/1
  [Iload] -> "Power (3ph, Phasor)1"/2
  [Igrid] -> "Power (3ph, Phasor)"/2
  Bus Selector2/1 -> "to kW "/1  "<Pbatt>"
  [Vgrid] -> "Power (3ph, Phasor)"/1
  to kW/1 -> Scope1/2, Bus Creator/1  "PV"
  "Power (3ph, Phasor)"/1 -> to  kW/1
  "Power (3ph, Phasor)1"/1 -> " to kW"/1
  to  kW/1 -> Bus Creator/3  "Grid"
  Bus Selector1/1 -> SOC (%)/1  "ESS State of Charge (%)"
  Bus Selector3/2 -> <PV>/1  "<PV>"
  Bus Selector3/1 -> <Load>/1  "<Load>"
  [battM] -> Bus Selector1/1, Bus Selector2/1
  [distP] -> Bus Selector/1
  Bus Selector/1 -> Gain/1  "<Grid>"
  Integrator/1 -> Scope/1  "Grid Usage"
  Gain/1 -> Integrator/1
  Demux1/4 -> Energy (kWh)/4  "Load"
  Demux1/3 -> Energy (kWh)/3  "PV"
  to kWh/1 -> Demux1/1
  Demux1/2 -> Energy (kWh)/2  "BESS"
  Integrator1/1 -> to kWh/1
  Demux1/1 -> Energy (kWh)/1  "Grid"

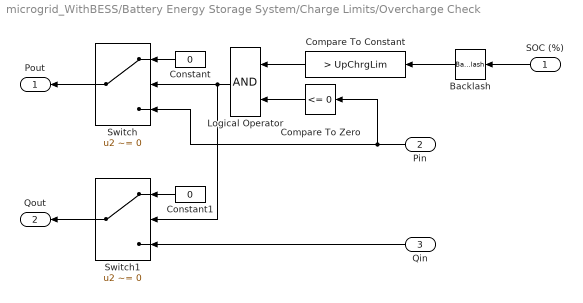
== system microgrid_WithBESS/Battery Energy Storage System/Charge Limits/Overcharge Check ==
  SOC (%) : Inport
  Pin : Inport  Port=2
  Qin : Inport  Port=3
  Backlash : Backlash  BacklashWidth=1e-3  InitialOutput=Initial_kWh_pc  ZeroCross=off
  Compare To Constant : simulink/Logic and Bit Operations/Compare To Constant  relop=>  const=UpChrgLim  OutDataTypeStr=boolean
  Compare To Zero : simulink/Logic and Bit Operations/Compare To Zero  relop=<=  OutDataTypeStr=boolean
  Constant : Constant  Value=0
  Constant1 : Constant  Value=0
  Logical Operator : Logic  AllPortsSameDT=off  OutDataTypeStr=boolean
  Switch : Switch  Criteria=u2 ~= 0  SaturateOnIntegerOverflow=off  InputSameDT=off
  Switch1 : Switch  Criteria=u2 ~= 0  SaturateOnIntegerOverflow=off  InputSameDT=off
  Pout : Outport  VectorParamsAs1DForOutWhenUnconnected=off
  Qout : Outport  Port=2  VectorParamsAs1DForOutWhenUnconnected=off
  wires:
  Backlash/1 -> Compare To Constant/1
  Switch1/1 -> Qout/1
  Constant1/1 -> Switch1/1
  Qin/1 -> Switch1/3
  Compare To Zero/1 -> Logical Operator/2
  Switch/1 -> Pout/1
  Pin/1 -> Switch/3, Compare To Zero/1
  SOC (%)/1 -> Backlash/1
  Constant/1 -> Switch/1
  Logical Operator/1 -> Switch/2, Switch1/2
  Compare To Constant/1 -> Logical Operator/1

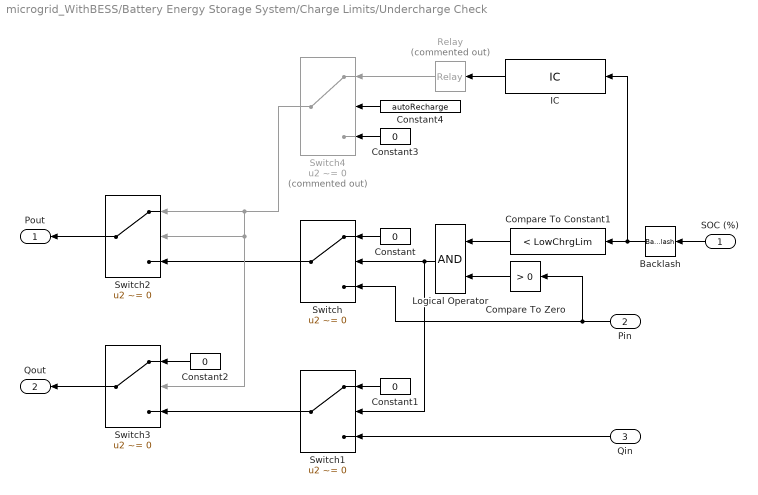
== system microgrid_WithBESS/Battery Energy Storage System/Charge Limits/Undercharge Check ==
  SOC (%) : Inport
  Pin : Inport  Port=2
  Qin : Inport  Port=3
  Backlash : Backlash  BacklashWidth=1e-3  InitialOutput=Initial_kWh_pc  ZeroCross=off
  Compare To Constant1 : simulink/Logic and Bit Operations/Compare To Constant  relop=<  const=LowChrgLim  OutDataTypeStr=boolean
  Compare To Zero : simulink/Logic and Bit Operations/Compare To Zero  relop=>  OutDataTypeStr=boolean
  Constant{,1..3} (4 alike) : Constant  Value=0
  Constant4 : Constant  Value=autoRecharge
  IC : InitialCondition  Value=RechargeSOC
  Logical Operator : Logic  AllPortsSameDT=off  OutDataTypeStr=boolean
  Relay : Relay  Commented=on  OnSwitchValue=RechargeSOC  OffSwitchValue=LowChrgLim  OnOutputValue=0  OffOutputValue=-Precharge/100*Pnom
  Switch{,1..3} (4 alike) : Switch  Criteria=u2 ~= 0  SaturateOnIntegerOverflow=off  InputSameDT=off
  Switch4 : Switch  Commented=on  Criteria=u2 ~= 0  SaturateOnIntegerOverflow=off  InputSameDT=off
  Pout : Outport  VectorParamsAs1DForOutWhenUnconnected=off
  Qout : Outport  Port=2  VectorParamsAs1DForOutWhenUnconnected=off
  wires:
  Constant4/1 -> Switch4/2
  Constant3/1 -> Switch4/3
  Relay/1 -> Switch4/1
  Constant2/1 -> Switch3/1
  Switch1/1 -> Switch3/3
  Switch3/1 -> Qout/1
  Switch2/1 -> Pout/1
  Switch/1 -> Switch2/3
  IC/1 -> Relay/1
  Switch4/1 -> Switch3/2, Switch2/2, Switch2/1
  Backlash/1 -> Compare To Constant1/1, IC/1
  Qin/1 -> Switch1/3
  Constant1/1 -> Switch1/1
  Compare To Constant1/1 -> Logical Operator/1
  Logical Operator/1 -> Switch1/2, Switch/2
  Constant/1 -> Switch/1
  SOC (%)/1 -> Backlash/1
  Pin/1 -> Compare To Zero/1, Switch/3
  Compare To Zero/1 -> Logical Operator/2

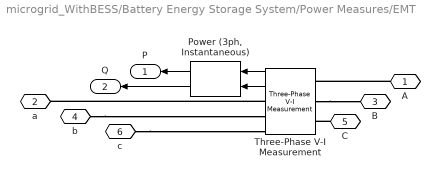
== system microgrid_WithBESS/Battery Energy Storage System/Power Measures/EMT ==
  "Power (3ph, Instantaneous)" : powerlib_meascontrol/Measurements/Power (3ph, Instantaneous)
  Three-Phase V-I Measurement : powerlib/Measurements/Three-Phase V-I Measurement  VoltageMeasurement=phase-to-ground  SetLabelV=off  LabelV=Vabc  Vpu=off  VpuLL=off  CurrentMeasurement=yes  SetLabelI=off  LabelI=Iabc  Ipu=off  Pbase=100e6  Vbase=500e3  OutputType=Complex  PhasorSimulation=on  PSBequivalent=0
  A : PMIOPort  Side=Left
  a : PMIOPort  Port=2  Side=Right
  B : PMIOPort  Port=3  Side=Left
  b : PMIOPort  Port=4  Side=Right
  C : PMIOPort  Port=5  Side=Left
  c : PMIOPort  Port=6  Side=Right
  P : Outport  VectorParamsAs1DForOutWhenUnconnected=off
  Q : Outport  Port=2  VectorParamsAs1DForOutWhenUnconnected=off
  wires:
  Three-Phase V-I Measurement/2 -> "Power (3ph, Instantaneous)"/2
  Three-Phase V-I Measurement/1 -> "Power (3ph, Instantaneous)"/1
  "Power (3ph, Instantaneous)"/1 -> P/1
  "Power (3ph, Instantaneous)"/2 -> Q/1
  connections:
  Three-Phase V-I Measurement/RConn1 -- a/RConn1
  b/RConn1 -- Three-Phase V-I Measurement/RConn2
  A/RConn1 -- Three-Phase V-I Measurement/LConn1
  Three-Phase V-I Measurement/LConn2 -- B/RConn1
  c/RConn1 -- Three-Phase V-I Measurement/RConn3
  C/RConn1 -- Three-Phase V-I Measurement/LConn3

== system microgrid_WithBESS/Battery Energy Storage System/Power Measures/Phasor ==
  "Power (3ph, Phasor)" : spsPower3phPhasorLib/Power (3ph, Phasor)
      settings: LibrarySourceBlock=|
      | sps_lib/Sensors and Measurements/Power
      | (3ph, Phasor)
  Three-Phase V-I Measurement : spsThreePhaseVIMeasurementLib/Three-Phase V-I Measurement  VoltageMeasurement=phase-to-ground  SetLabelV=off  LabelV=Vabc  Vpu=off  VpuLL=off  CurrentMeasurement=yes  SetLabelI=off  LabelI=Iabc  Ipu=off  Pbase=100e6  Vbase=500e3  OutputType=Complex  PhasorSimulation=on  PSBequivalent=0
  A : PMIOPort  Side=Left
  a : PMIOPort  Port=2  Side=Right
  B : PMIOPort  Port=3  Side=Left
  b : PMIOPort  Port=4  Side=Right
  C : PMIOPort  Port=5  Side=Left
  c : PMIOPort  Port=6  Side=Right
  P : Outport  VectorParamsAs1DForOutWhenUnconnected=off
  Q : Outport  Port=2  VectorParamsAs1DForOutWhenUnconnected=off
  wires:
  "Power (3ph, Phasor)"/2 -> Q/1
  "Power (3ph, Phasor)"/1 -> P/1
  Three-Phase V-I Measurement/1 -> "Power (3ph, Phasor)"/1
  Three-Phase V-I Measurement/2 -> "Power (3ph, Phasor)"/2
  connections:
  C/RConn1 -- Three-Phase V-I Measurement/LConn3
  c/RConn1 -- Three-Phase V-I Measurement/RConn3
  Three-Phase V-I Measurement/LConn2 -- B/RConn1
  A/RConn1 -- Three-Phase V-I Measurement/LConn1
  b/RConn1 -- Three-Phase V-I Measurement/RConn2
  Three-Phase V-I Measurement/RConn1 -- a/RConn1

== system microgrid_WithBESS/Energy Management System/24 Hour Clock/Enabled Subsystem ==
  In1 : Inport
  Enable : EnablePort
  Out1 : Outport  VectorParamsAs1DForOutWhenUnconnected=off
  wires:
  In1/1 -> Out1/1

== matlab function microgrid_WithBESS/Energy Management System/Linear Programming Optimization Routine/Optimization-based Energy Management ==
  data: SOC input; optVec output size=1; Ebatt input; dt input; Cost input; Ppv input; Pload input
function optVec  = fcn(SOC,Ebatt,dt,Cost,Ppv,Pload)
%#codegen

M = 241;
optVec = 0;
Pbatt = zeros(M,1);
EnergyWeight = 1;

% Energy constraints
batteryMinMax.Emax = 0.8*Ebatt;
batteryMinMax.Emin = 0.2*Ebatt;

% Power constraints
batteryMinMax.Pmin = -143e3;
batteryMinMax.Pmax = 143e3;

% Declare function (contains linprog) as extrinsic
coder.extrinsic('battSolarOptimize');

% Battery parameters
Einit = SOC/100*Ebatt;

[~,Pbatt,~] = battSolarOptimize(M,dt,Ppv,Pload,Einit,Cost,...
    EnergyWeight,batteryMinMax);

optVec = Pbatt(1);
% optVec = mean(Pbatt(1:5));

== stateflow chart microgrid_WithBESS/Energy Management System/Chart ==
  state disableBESS
    Pcmd = 0;
  state BMS
    state IdleBESS
      Pcmd = 0;
      state MPPTOff
      state LoadShedding
      (default) -> BMS.IdleBESS.MPPTOff
      BMS.IdleBESS.MPPTOff -> BMS.IdleBESS.LoadShedding : [SOC <= minSOC]
      BMS.IdleBESS.LoadShedding -> BMS.IdleBESS.MPPTOff : [SOC >= maxSOC]
    state PeakSupply
      Pcmd = Pmax;
    state NightRecharge
      Pcmd = Pmin;
    state AbsorbSupplyPV
      Pnet = 1e3*(Load-PV);
      state Discharging
        Pcmd= Pnet;
      state Charging
        Pcmd = Pnet;
      state MPPTOff
        Pcmd = Pmin;
      state LoadShedding
        Pcmd = Pmax;
      (default) -> Charging
      Charging -> Discharging [order 1] : [Load> PV]
      Discharging -> Charging [order 1] : [Load< PV]
      Charging -> BMS.AbsorbSupplyPV.MPPTOff [order 2] : [Pnet < Pmin]
      BMS.AbsorbSupplyPV.MPPTOff -> Charging : [Pnet > Pmin]
      Discharging -> BMS.AbsorbSupplyPV.LoadShedding [order 2] : [Pnet > Pmax]
      BMS.AbsorbSupplyPV.LoadShedding -> Discharging : [Pnet < Pmax]
    (default) -> IdleBESS
    PeakSupply -> NightRecharge : [Time > 23]
    IdleBESS -> PeakSupply [order 2] : [Time > 18]
    NightRecharge -> (junction 97)
    (junction 95) -> IdleBESS
    (junction 97) -> (junction 95) : [SOC >= maxSOC]
    AbsorbSupplyPV -> (junction 95) : [SOC >= maxSOC ...
        |   || SOC <= minSOC]
    IdleBESS -> (junction 102) [order 1] : [Time > 6 && Time < 15]
    (junction 102) -> AbsorbSupplyPV : [SOC > minSOC && SOC < maxSOC]
  (default) -> disableBESS
  disableBESS -> BMS : [ESS == 1]
  data: Pcmd output; Load input; PV input; SOC input; maxSOC constant double =80; minSOC constant double =20; Pmax constant double =1e3*400; Pmin constant double =-1e3*400; Pnet local; ESS input; Time input
